simulink model "bouncing"  (Simulink 7.9)
settings: Solver=ode45  StartTime=0.0  StopTime=10.0  RelTol=1e-3
libraries: vrlib x1
settings Model: Creator=prakrit  LastModifiedBy=prakrit

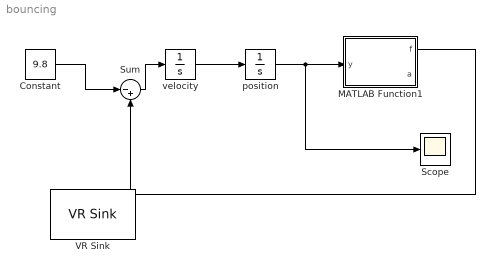
== system bouncing ==
  Constant : Constant  Value=9.8
  MATLAB Function1 : MATLAB Function  TreatAsAtomicUnit=on
  Scope : Scope
  Sum : Sum  Inputs=|-+
  VR Sink : vrlib/VR Sink  SampleTime=0.1  ViewEnable=on  RemoteChange=off  RemoteView=on  AutoView=off  VideoDimensions=[]  AllowVariableSize=off
  position : Integrator  InitialCondition=20
  velocity : Integrator
  wires:
  velocity/1 -> position/1
  position/1 -> MATLAB Function1/1(y), Scope/1
  Constant/1 -> Sum/1
  Sum/1 -> velocity/1
  MATLAB Function1/1(f) -> Sum/2

== matlab function MATLAB Function1 ==
  data: y input double; f output double; a output double
function [f,a] = fcn(y)

if y<1e-4
    y=1e-4;
end
if y<1.5
    f = 500*(1.5-y);
    a = sqrt(1.5^3/y);
else
    f = 0;
    a = 1.5;
end
